simulink model "task3"  (R2022b)
settings: Solver=VariableStepAuto  StartTime=0.0  StopTime=2  RelTol=1e-3
settings Model: Creator=af063  LastModifiedBy=af063

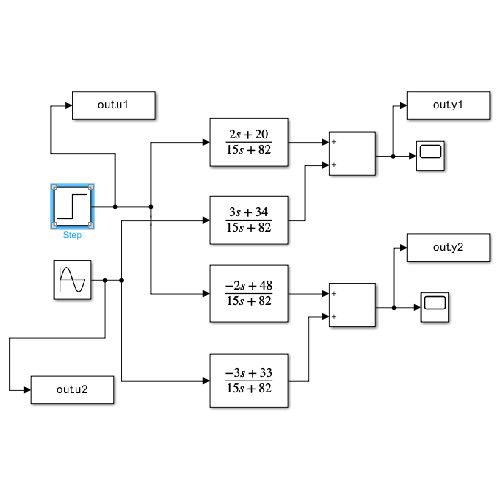
[thumbnail: Simulink's stored preview of the top-level diagram]
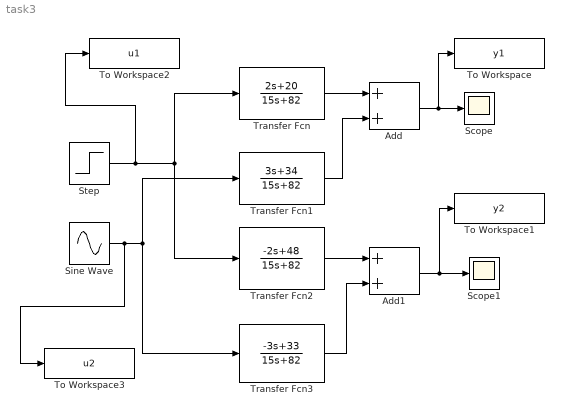
== system task3 ==
  Add : Sum
  Add1 : Sum
  Scope : Scope
  Scope1 : Scope
  Sine Wave : Sin  Amplitude=2  SampleTime=0
  Step : Step  Time=0  SampleTime=0
  To Workspace : ToWorkspace  VariableName=y1  SampleTime=-1
  To Workspace1 : ToWorkspace  VariableName=y2  SampleTime=-1
  To Workspace2 : ToWorkspace  VariableName=u1  SampleTime=-1
  To Workspace3 : ToWorkspace  VariableName=u2  SampleTime=-1
  Transfer Fcn : TransferFcn  Numerator=[2 20]  Denominator=[15 82]
  Transfer Fcn1 : TransferFcn  Numerator=[3 34]  Denominator=[15 82]
  Transfer Fcn2 : TransferFcn  Numerator=[-2 48]  Denominator=[15 82]
  Transfer Fcn3 : TransferFcn  Numerator=[-3 33]  Denominator=[15 82]
  wires:
  Step/1 -> To Workspace2/1, Transfer Fcn2/1, Transfer Fcn/1
  Sine Wave/1 -> To Workspace3/1, Transfer Fcn3/1, Transfer Fcn1/1
  Transfer Fcn/1 -> Add/1
  Transfer Fcn1/1 -> Add/2
  Transfer Fcn2/1 -> Add1/1
  Transfer Fcn3/1 -> Add1/2
  Add/1 -> To Workspace/1, Scope/1
  Add1/1 -> To Workspace1/1, Scope1/1
